simulink model "controller_8_9_2021_final"  (R2021a)
settings: Solver=ode23t  StartTime=0.0  StopTime=1.3  MaxStep=1  RelTol=1e-3  AbsTol=1e-3
model workspace (MAT data in the model file):
  T_ret = 0.5547
  T_standby = 0.2
values from neighbouring files (symbols this model uses):
  calculated_T_ramp = 0.012    [catapultScript_8_9_2021_final.m]
  calculated_T_ret = 0.07    [catapultScript_8_9_2021_final.m]
  calculated_W_cruise = 17.0    (= 17)    [catapultScript_8_9_2021_final.m]
  markerPosition = X_TARGET + L    [catapultScript_8_9_2021_final.m]
  speed_I = 1.2    [catapultScript_8_9_2021_final.m]
  speed_P = 2.6    [catapultScript_8_9_2021_final.m]
undefined symbols (not defined in the file or in its folder): ballNumber, torque, X, Y, Z
libraries: sm_lib x33, nesl_utility x11, ee_lib x6, fl_lib x5, pid_lib x2
(part 2 of 2)

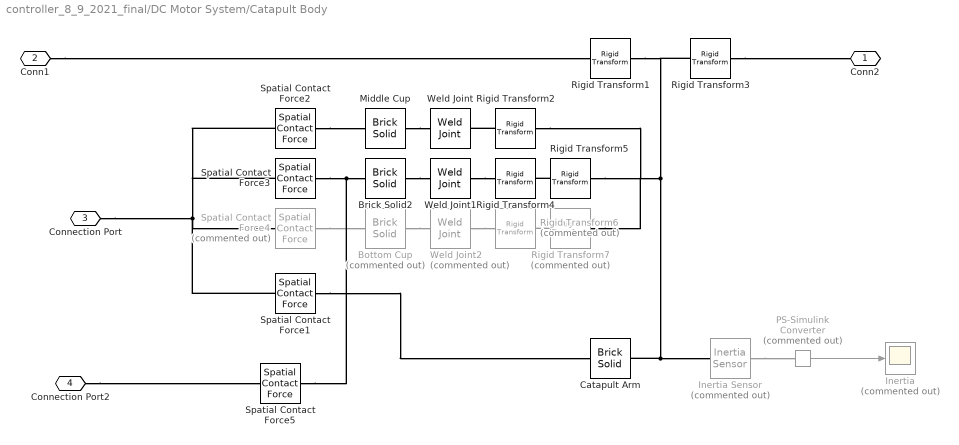
== system controller_8_9_2021_final/DC Motor System/Catapult Body ==
  Bottom Cup : sm_lib/Body Elements/Brick Solid  Commented=on  GraphicAmbientColor=[0.15 0.15 0.15 1.0]  BasedOnType=Density  BrickDimensions=[6 3 0.5]  BrickDimensionUnits=cm  CenterOfMass=[0 0 0]  CenterOfMassUnits=m  GraphicDiffuseColor=[0.0 0.8 0.6]  Density=1100  DensityUnits=kg/m^3  DoExposeReferenceFrame=on  GraphicEmissiveColor=[0.0 0.0 0.0 1.0]  ExportEntireGeometry=on  SerializedFrames=<Frames/>  MarkerShape=Sphere  MarkerSize=10  GraphicType=FromGeometry  InertiaType=CalculateFromGeometry  Mass=0  MassUnits=kg  MomentsOfInertia=[1 1 1]  MomentsOfInertiaUnits=kg*m^2  GraphicOpacity=1.0  ProductsOfInertia=[0 0 0]  ProductsOfInertiaUnits=kg*m^2  GraphicShininess=75  GraphicSpecularColor=[0.5 0.5 0.5 1.0]  GraphicVisPropType=SimpleVisualProperties
  Brick Solid2 : sm_lib/Body Elements/Brick Solid  GraphicAmbientColor=[0.15 0.15 0.15 1.0]  BasedOnType=Density  BrickDimensions=[6 3.5 0.5]  BrickDimensionUnits=cm  CenterOfMass=[0 0 0]  CenterOfMassUnits=m  GraphicDiffuseColor=[0.0 0.8 0.6]  Density=1100  DensityUnits=kg/m^3  DoExposeReferenceFrame=on  GraphicEmissiveColor=[0.0 0.0 0.0 1.0]  ExportEntireGeometry=on  SerializedFrames=<Frames/>  MarkerShape=Sphere  MarkerSize=10  GraphicType=FromGeometry  InertiaType=CalculateFromGeometry  Mass=1  MassUnits=kg  MomentsOfInertia=[1 1 1]  MomentsOfInertiaUnits=kg*m^2  GraphicOpacity=1.0  ProductsOfInertia=[0 0 0]  ProductsOfInertiaUnits=kg*m^2  GraphicShininess=75  GraphicSpecularColor=[0.5 0.5 0.5 1.0]  GraphicVisPropType=SimpleVisualProperties
  Catapult Arm : sm_lib/Body Elements/Brick Solid  GraphicAmbientColor=[0.15 0.15 0.15 1.0]  BasedOnType=Density  BrickDimensions=[27 2 2]  BrickDimensionUnits=cm  CenterOfMass=[0 0 0]  CenterOfMassUnits=m  GraphicDiffuseColor=[0.0 0.8 0.8]  Density=1100  DensityUnits=kg/m^3  DoExposeReferenceFrame=on  GraphicEmissiveColor=[0.0 0.0 0.0 1.0]  ExportEntireGeometry=on  SerializedFrames=<Frames/>  MarkerShape=Sphere  MarkerSize=10  GraphicType=FromGeometry  InertiaType=CalculateFromGeometry  Mass=1  MassUnits=kg  MomentsOfInertia=[2.291563*10^-3 0 0]  MomentsOfInertiaUnits=kg*m^2  GraphicOpacity=1.0  ProductsOfInertia=[0 0 0]  ProductsOfInertiaUnits=kg*m^2  GraphicShininess=75  GraphicSpecularColor=[0.5 0.5 0.5 1.0]  GraphicVisPropType=SimpleVisualProperties
  Inertia : Scope  Commented=on
  Inertia Sensor : sm_lib/Body Elements/Inertia Sensor  Commented=on  SensorExtent=BodyGroup  SpanWeldJoints=on  ExcludeGroundedBodies=off  MeasurementFrame=Attached  SenseMass=off  SenseCenterOfMass=off  SenseInertiaMatrix=off  SenseCenteredInertiaMatrix=off  SensePrincipalInertiaMatrix=on  SenseRotationMatrix=off  GraphicType=PrincipalInertiaFrame  PrincipalInertiaFrameSize=20  GraphicVisPropType=SimpleVisualProperties  GraphicDiffuseColor=[0.5 0.5 0.5]  GraphicSpecularColor=[0.5 0.5 0.5 1.0]  GraphicAmbientColor=[0.15 0.15 0.15 1.0]  GraphicEmissiveColor=[0.0 0.0 0.0 1.0]  GraphicShininess=75  GraphicOpacity=1.0
      settings: SourceProductBaseCode=MS
  Middle Cup : sm_lib/Body Elements/Brick Solid  GraphicAmbientColor=[0.15 0.15 0.15 1.0]  BasedOnType=Density  BrickDimensions=[6 6 1]  BrickDimensionUnits=cm  CenterOfMass=[0 0 0]  CenterOfMassUnits=m  GraphicDiffuseColor=[0.0 0.8 0.6]  Density=1100  DensityUnits=kg/m^3  DoExposeReferenceFrame=on  GraphicEmissiveColor=[0.0 0.0 0.0 1.0]  ExportEntireGeometry=on  SerializedFrames=<Frames/>  MarkerShape=Sphere  MarkerSize=10  GraphicType=FromGeometry  InertiaType=CalculateFromGeometry  Mass=1  MassUnits=kg  MomentsOfInertia=[1 1 1]  MomentsOfInertiaUnits=kg*m^2  GraphicOpacity=1.0  ProductsOfInertia=[0 0 0]  ProductsOfInertiaUnits=kg*m^2  GraphicShininess=75  GraphicSpecularColor=[0.5 0.5 0.5 1.0]  GraphicVisPropType=SimpleVisualProperties
  PS-Simulink Converter : nesl_utility/PS-Simulink Converter  Commented=on  PhysicalDomain=network_engine_domain  SubClassName=ps_output  LeftPortType=input  RightPortType=output  PseudoPeriodic=off  Frequencies=[]  Unit=inherit  AffineConversion=off
      settings: SourceProductBaseCode=PW,SS
  Rigid Transform1 : sm_lib/Frames and Transforms/Rigid Transform  TranslationMethod=StandardAxis  TranslationStandardOffset=-13.5  TranslationLengthUnit=cm  TranslationStandardAxis=+X  TranslationCartesianOffset=[0 0 0]  TranslationROffset=0  TranslationROffsetUnits=m  TranslationZOffset=0  TranslationZOffsetUnits=m  TranslationThetaOffset=0  TranslationThetaOffsetUnits=deg  RotationMethod=StandardAxis  RotationAngleUnits=deg  RotationStandardAxis=+Z  RotationAngle=forcedArmAngle  RotationArbitraryAxis=[0 0 1]  FollAlignAxisA=+X  BaseAlignAxisA=+Y  FollAlignAxisB=+Y  BaseAlignAxisB=+Z  RotationSequenceAxes=FollowerAxes  RotationSequence=XYX  RotationSequenceAngles=[0 0 0]  RotationSequenceAnglesUnits=deg  RotationMatrix=[1 0 0; 0 1 0; 0 0 1]
  Rigid Transform2 : sm_lib/Frames and Transforms/Rigid Transform  TranslationMethod=Cartesian  TranslationStandardOffset=7  TranslationLengthUnit=cm  TranslationStandardAxis=-X  TranslationCartesianOffset=[-11 0 -1]  TranslationROffset=0  TranslationROffsetUnits=m  TranslationZOffset=0  TranslationZOffsetUnits=m  TranslationThetaOffset=0  TranslationThetaOffsetUnits=deg  RotationMethod=StandardAxis  RotationAngleUnits=deg  RotationStandardAxis=+X  RotationAngle=90  RotationArbitraryAxis=[0 0 1]  FollAlignAxisA=+X  BaseAlignAxisA=+Y  FollAlignAxisB=+Y  BaseAlignAxisB=+Z  RotationSequenceAxes=FollowerAxes  RotationSequence=XYX  RotationSequenceAngles=[90 0 0]  RotationSequenceAnglesUnits=deg  RotationMatrix=[1 0 0; 0 1 0; 0 0 1]
  Rigid Transform3 : sm_lib/Frames and Transforms/Rigid Transform  TranslationMethod=StandardAxis  TranslationStandardOffset=7  TranslationLengthUnit=cm  TranslationStandardAxis=+X  TranslationCartesianOffset=[0 0 0]  TranslationROffset=0  TranslationROffsetUnits=m  TranslationZOffset=0  TranslationZOffsetUnits=m  TranslationThetaOffset=0  TranslationThetaOffsetUnits=deg  RotationMethod=None  RotationAngleUnits=deg  RotationStandardAxis=+Z  RotationAngle=30  RotationArbitraryAxis=[0 0 1]  FollAlignAxisA=+X  BaseAlignAxisA=+Y  FollAlignAxisB=+Y  BaseAlignAxisB=+Z  RotationSequenceAxes=FollowerAxes  RotationSequence=XYX  RotationSequenceAngles=[0 0 0]  RotationSequenceAnglesUnits=deg  RotationMatrix=[1 0 0; 0 1 0; 0 0 1]
  Rigid Transform4 : sm_lib/Frames and Transforms/Rigid Transform  TranslationMethod=Cartesian  TranslationStandardOffset=7  TranslationLengthUnit=cm  TranslationStandardAxis=-X  TranslationCartesianOffset=[-7 0 -1]  TranslationROffset=0  TranslationROffsetUnits=m  TranslationZOffset=0  TranslationZOffsetUnits=m  TranslationThetaOffset=0  TranslationThetaOffsetUnits=deg  RotationMethod=StandardAxis  RotationAngleUnits=deg  RotationStandardAxis=+X  RotationAngle=90  RotationArbitraryAxis=[0 0 1]  FollAlignAxisA=+X  BaseAlignAxisA=+Y  FollAlignAxisB=+Y  BaseAlignAxisB=+Z  RotationSequenceAxes=FollowerAxes  RotationSequence=XYX  RotationSequenceAngles=[90 0 0]  RotationSequenceAnglesUnits=deg  RotationMatrix=[1 0 0; 0 1 0; 0 0 1]
  Rigid Transform5 : sm_lib/Frames and Transforms/Rigid Transform  TranslationMethod=Cartesian  TranslationStandardOffset=7  TranslationLengthUnit=cm  TranslationStandardAxis=-X  TranslationCartesianOffset=[7 -13.2 -4]  TranslationROffset=0  TranslationROffsetUnits=m  TranslationZOffset=0  TranslationZOffsetUnits=m  TranslationThetaOffset=0  TranslationThetaOffsetUnits=deg  RotationMethod=RotationSequence  RotationAngleUnits=deg  RotationStandardAxis=+X  RotationAngle=90  RotationArbitraryAxis=[0 0 1]  FollAlignAxisA=+X  BaseAlignAxisA=+Y  FollAlignAxisB=+Y  BaseAlignAxisB=+Z  RotationSequenceAxes=FollowerAxes  RotationSequence=XYX  RotationSequenceAngles=[90 90 0]  RotationSequenceAnglesUnits=deg  RotationMatrix=[1 0 0; 0 1 0; 0 0 1]
  Rigid Transform6 : sm_lib/Frames and Transforms/Rigid Transform  Commented=on  TranslationMethod=Cartesian  TranslationStandardOffset=7  TranslationLengthUnit=cm  TranslationStandardAxis=-X  TranslationCartesianOffset=[-7 0 -1]  TranslationROffset=0  TranslationROffsetUnits=m  TranslationZOffset=0  TranslationZOffsetUnits=m  TranslationThetaOffset=0  TranslationThetaOffsetUnits=deg  RotationMethod=StandardAxis  RotationAngleUnits=deg  RotationStandardAxis=+X  RotationAngle=90  RotationArbitraryAxis=[0 0 1]  FollAlignAxisA=+X  BaseAlignAxisA=+Y  FollAlignAxisB=+Y  BaseAlignAxisB=+Z  RotationSequenceAxes=FollowerAxes  RotationSequence=XYX  RotationSequenceAngles=[90 0 0]  RotationSequenceAnglesUnits=deg  RotationMatrix=[1 0 0; 0 1 0; 0 0 1]
  Rigid Transform7 : sm_lib/Frames and Transforms/Rigid Transform  Commented=on  TranslationMethod=Cartesian  TranslationStandardOffset=7  TranslationLengthUnit=cm  TranslationStandardAxis=-X  TranslationCartesianOffset=[7 -2.4 -4]  TranslationROffset=0  TranslationROffsetUnits=m  TranslationZOffset=0  TranslationZOffsetUnits=m  TranslationThetaOffset=0  TranslationThetaOffsetUnits=deg  RotationMethod=RotationSequence  RotationAngleUnits=deg  RotationStandardAxis=+X  RotationAngle=90  RotationArbitraryAxis=[0 0 1]  FollAlignAxisA=+X  BaseAlignAxisA=+Y  FollAlignAxisB=+Y  BaseAlignAxisB=+Z  RotationSequenceAxes=FollowerAxes  RotationSequence=XYX  RotationSequenceAngles=[90 90 0]  RotationSequenceAnglesUnits=deg  RotationMatrix=[1 0 0; 0 1 0; 0 0 1]
  Spatial Contact Force1 : sm_lib/Forces and Torques/Spatial Contact Force  CoefficientOfDynamicFriction=0.3  CoefficientOfStaticFriction=0.5  SenseContactBaseRotation=off  SenseContactBaseTranslation=off  NormalDamping=1e3  NormalDampingUnits=N/(m/s)  SenseContactFollowerRotation=off  SenseContactFollowerTranslation=off  SenseContactSignal=off  NormalStiffness=1e6  NormalStiffnessUnits=N/m  FrictionalCriticalVelocity=1e-3  FrictionalCriticalVelocityUnits=m/s  ZeroCrossDetectContactStartAndEnd=off  FrictionType=SmoothStickSlip  SenseFrictionalForceMagnitude=off  SenseNormalForceMagnitude=off  NormalForceType=SmoothSpringDamper  SenseNormalVelocity=off  SenseSeparationDistance=off  SenseTangentialVelocity=off  SenseTangentialVelocityMagnitude=off  NormalTransitionRegionWidth=1e-4  NormalTransitionRegionWidthUnits=m
  Spatial Contact Force2 : sm_lib/Forces and Torques/Spatial Contact Force  CoefficientOfDynamicFriction=0.3  CoefficientOfStaticFriction=0.5  SenseContactBaseRotation=off  SenseContactBaseTranslation=off  NormalDamping=1e3  NormalDampingUnits=N/(m/s)  SenseContactFollowerRotation=off  SenseContactFollowerTranslation=off  SenseContactSignal=off  NormalStiffness=1e6  NormalStiffnessUnits=N/m  FrictionalCriticalVelocity=1e-3  FrictionalCriticalVelocityUnits=m/s  ZeroCrossDetectContactStartAndEnd=off  FrictionType=None  SenseFrictionalForceMagnitude=off  SenseNormalForceMagnitude=off  NormalForceType=SmoothSpringDamper  SenseNormalVelocity=off  SenseSeparationDistance=off  SenseTangentialVelocity=off  SenseTangentialVelocityMagnitude=off  NormalTransitionRegionWidth=1e-4  NormalTransitionRegionWidthUnits=m
  Spatial Contact Force3 : sm_lib/Forces and Torques/Spatial Contact Force  CoefficientOfDynamicFriction=0.3  CoefficientOfStaticFriction=0.5  SenseContactBaseRotation=off  SenseContactBaseTranslation=off  NormalDamping=1e3  NormalDampingUnits=N/(m/s)  SenseContactFollowerRotation=off  SenseContactFollowerTranslation=off  SenseContactSignal=off  NormalStiffness=1e6  NormalStiffnessUnits=N/m  FrictionalCriticalVelocity=1e-3  FrictionalCriticalVelocityUnits=m/s  ZeroCrossDetectContactStartAndEnd=off  FrictionType=None  SenseFrictionalForceMagnitude=off  SenseNormalForceMagnitude=off  NormalForceType=SmoothSpringDamper  SenseNormalVelocity=off  SenseSeparationDistance=off  SenseTangentialVelocity=off  SenseTangentialVelocityMagnitude=off  NormalTransitionRegionWidth=1e-4  NormalTransitionRegionWidthUnits=m
  Spatial Contact Force4 : sm_lib/Forces and Torques/Spatial Contact Force  Commented=on  CoefficientOfDynamicFriction=0.3  CoefficientOfStaticFriction=0.5  SenseContactBaseRotation=off  SenseContactBaseTranslation=off  NormalDamping=1e3  NormalDampingUnits=N/(m/s)  SenseContactFollowerRotation=off  SenseContactFollowerTranslation=off  SenseContactSignal=off  NormalStiffness=1e6  NormalStiffnessUnits=N/m  FrictionalCriticalVelocity=1e-3  FrictionalCriticalVelocityUnits=m/s  ZeroCrossDetectContactStartAndEnd=off  FrictionType=SmoothStickSlip  SenseFrictionalForceMagnitude=off  SenseNormalForceMagnitude=off  NormalForceType=SmoothSpringDamper  SenseNormalVelocity=off  SenseSeparationDistance=off  SenseTangentialVelocity=off  SenseTangentialVelocityMagnitude=off  NormalTransitionRegionWidth=1e-4  NormalTransitionRegionWidthUnits=m
  Spatial Contact Force5 : sm_lib/Forces and Torques/Spatial Contact Force  CoefficientOfDynamicFriction=0.3  CoefficientOfStaticFriction=0.5  SenseContactBaseRotation=off  SenseContactBaseTranslation=off  NormalDamping=1e3  NormalDampingUnits=N/(m/s)  SenseContactFollowerRotation=off  SenseContactFollowerTranslation=off  SenseContactSignal=off  NormalStiffness=1e6  NormalStiffnessUnits=N/m  FrictionalCriticalVelocity=1e-3  FrictionalCriticalVelocityUnits=m/s  ZeroCrossDetectContactStartAndEnd=off  FrictionType=SmoothStickSlip  SenseFrictionalForceMagnitude=off  SenseNormalForceMagnitude=off  NormalForceType=SmoothSpringDamper  SenseNormalVelocity=off  SenseSeparationDistance=off  SenseTangentialVelocity=off  SenseTangentialVelocityMagnitude=off  NormalTransitionRegionWidth=1e-4  NormalTransitionRegionWidthUnits=m
  Weld Joint : sm_lib/Joints/Weld Joint  JointMode=Normal  SenseConstraintForce=off  SenseConstraintForceX=off  SenseConstraintForceY=off  SenseConstraintForceZ=off  SenseConstraintTorque=off  SenseConstraintTorqueX=off  SenseConstraintTorqueY=off  SenseConstraintTorqueZ=off  SenseTotalForce=off  SenseTotalForceX=off  SenseTotalForceY=off  SenseTotalForceZ=off  SenseTotalTorque=off  SenseTotalTorqueX=off  SenseTotalTorqueY=off  SenseTotalTorqueZ=off  CompositeWrenchDir=FollowerOnBase  CompositeWrenchFrame=BaseFrame
  Weld Joint1 : sm_lib/Joints/Weld Joint  JointMode=Normal  SenseConstraintForce=off  SenseConstraintForceX=off  SenseConstraintForceY=off  SenseConstraintForceZ=off  SenseConstraintTorque=off  SenseConstraintTorqueX=off  SenseConstraintTorqueY=off  SenseConstraintTorqueZ=off  SenseTotalForce=off  SenseTotalForceX=off  SenseTotalForceY=off  SenseTotalForceZ=off  SenseTotalTorque=off  SenseTotalTorqueX=off  SenseTotalTorqueY=off  SenseTotalTorqueZ=off  CompositeWrenchDir=FollowerOnBase  CompositeWrenchFrame=BaseFrame
  Weld Joint2 : sm_lib/Joints/Weld Joint  Commented=on  JointMode=Normal  SenseConstraintForce=off  SenseConstraintForceX=off  SenseConstraintForceY=off  SenseConstraintForceZ=off  SenseConstraintTorque=off  SenseConstraintTorqueX=off  SenseConstraintTorqueY=off  SenseConstraintTorqueZ=off  SenseTotalForce=off  SenseTotalForceX=off  SenseTotalForceY=off  SenseTotalForceZ=off  SenseTotalTorque=off  SenseTotalTorqueX=off  SenseTotalTorqueY=off  SenseTotalTorqueZ=off  CompositeWrenchDir=FollowerOnBase  CompositeWrenchFrame=BaseFrame
  Conn2 : PMIOPort  Side=Right
  Conn1 : PMIOPort  Port=2  Side=Left
  Connection Port : PMIOPort  Port=3  Side=Left
  Connection Port2 : PMIOPort  Port=4  Side=Left
  wires:
  PS-Simulink Converter/1 -> Inertia/1
  connections:
  Rigid Transform7/LConn1 -- Rigid Transform6/RConn1
  Weld Joint2/RConn1 -- Rigid Transform6/LConn1
  Bottom Cup/RConn1 -- Weld Joint2/LConn1
  Rigid Transform5/LConn1 -- Rigid Transform4/RConn1
  Weld Joint1/RConn1 -- Rigid Transform4/LConn1
  Brick Solid2/RConn1 -- Weld Joint1/LConn1
  Middle Cup/RConn1 -- Weld Joint/LConn1
  Spatial Contact Force1/RConn1 -- Catapult Arm/LConn1
  Rigid Transform3/LConn1 -- Conn2/RConn1
  Conn1/RConn1 -- Rigid Transform1/RConn1
  Rigid Transform7/RConn1 -- Rigid Transform5/RConn1 -- Rigid Transform2/RConn1 -- Rigid Transform1/LConn1 -- Rigid Transform3/RConn1 -- Catapult Arm/RConn1 -- Inertia Sensor/LConn1
  Rigid Transform2/LConn1 -- Weld Joint/RConn1
  Inertia Sensor/RConn1 -- PS-Simulink Converter/LConn1
  Connection Port/RConn1 -- Spatial Contact Force3/LConn1 -- Spatial Contact Force2/LConn1 -- Spatial Contact Force1/LConn1 -- Spatial Contact Force4/LConn1
  Spatial Contact Force4/RConn1 -- Bottom Cup/LConn1
  Spatial Contact Force3/RConn1 -- Spatial Contact Force5/RConn1 -- Brick Solid2/LConn1
  Spatial Contact Force2/RConn1 -- Middle Cup/LConn1
  Connection Port2/RConn1 -- Spatial Contact Force5/LConn1

== matlab function controller_8_9_2021_final/MATLAB Function ==
  data: t input; ballNumber input; T_standby input; controlSwitch output; stage0Done input; T_ramp input; T_ret input; T_fin input; W_cruise input; Q_ret input; S3_ACCEL input; q_d output; dq_d output; d2q_d output
%References
% https://www.mathworks.com/help/matlab/ref/function.html
% Dr. Moallem's code - checked inputs & outputs initially,used inverse method for the quintic controller, and compared
% sections of my written code with his



%do we want to use T_ret or Theta_ret to switch stage?

function [controlSwitch, q_d, dq_d, d2q_d] = catapult_control( t,ballNumber,T_standby,stage0Done,T_ramp, T_ret, T_fin, W_cruise, Q_ret,S3_ACCEL) 
%function [controlSwitch, e_sc, e_pc, q_d, dq_d, d2q_d] = catapult_control( t,stage0Done,T_ramp, T_ret, T_fin, W_cruise, Q_ret, tau_scommand, tau_pcommand, theta, w, S3_ACCEL) 
%^ old header using tau,tau_scommand, tau_pcommand


controlSwitch = 0; %0 -> speed controller, 1 -> position controller

if stage0Done == 1
    t = t - T_standby;
end

%Stage 0 (Move to Starting Position: Q_ret)
% if stage0Done ~= 1 && t < T_standby && t < 0.8 && ballNumber == 1
%     %tau = tau_scommand; %based on speed control output
%     d2q_d = 2/0.8; %0.8s rise tarm hardcoded
%     dq_d = 2*t/0.8;
%      q_d = 0.5*d2q_d*(t^2);
%     %e_sc = dq_d - w;
%     %e_pc = 0; %since we don't need to change the system based on it
if stage0Done ~= 1 && t < T_standby
    controlSwitch = 1;
    q_d = Q_ret;
    dq_d = 0;
    d2q_d = 0;
    %e_sc = dq_d - w;
    %e_pc = q_d - theta;
    %tau = tau_pcommand;


%Stage 1 (Ramp up phase)
elseif t > 0 && t < T_ramp %Stage 1
controlSwitch = 0;    
    %tau = tau_scommand; %based on speed control output
    d2q_d = W_cruise/T_ramp;
    dq_d = W_cruise*t/T_ramp;
     q_d = 0.5*d2q_d*(t^2)+Q_ret;
    %e_sc = dq_d - w;
    %e_pc = 0; %since we don't need to change the system based on it

%Stage 2 (Constant Speed phase)
elseif t >= T_ramp && t < T_ret %Stage 2
    controlSwitch = 0;      
    %tau = tau_scommand; %based on speed control output
    q_d = 0.5*(W_cruise/T_ramp)*(T_ramp^2) + W_cruise*(t-T_ramp)+Q_ret; 
    dq_d = W_cruise;
    d2q_d = 0;
    %e_sc = W_cruise - w;
    %e_pc = 0; %since don't need to change the system based on it

 

%Stage 3 (Return Phase)
elseif t >= T_ret && t < T_fin %Stage 3
    controlSwitch = 1;   
    AT = T_fin - T_ret;
    %calculating qs
    q0 = 0.5*(W_cruise/T_ramp)*(T_ramp^2) + W_cruise*(T_ret - T_ramp)+Q_ret; %0.5*W_cruise*(T_ramp); %%It seems he already had the angle at this point known and hardcoded 

    q1 = W_cruise;
    q2 = 0.5*S3_ACCEL;
    
    ii= inv([AT^3 AT^4 AT^5; 3*AT^2 4*AT^3 5*AT^4; 6*AT 12*AT^2 20*AT^3])*[-(q0-Q_ret)-q1*AT-q2*AT^2; -q1-2*q2*AT; -2*q2];
    q3 = ii(1);
    q4 = ii(2);
    q5 = ii(3);
    %q5 = -(q0 + q1 - 0.3*q1*(T_fin - T_ret) - 0.6*q2*(T_fin - T_ret) + 1.033*q2*((T_fin - T_ret)^2))/(6.5*((T_fin - T_ret)^5));
    %q4 = -(q1 + 2*q2 + q2*((T_fin - T_ret) + 15*q5*((T_fin - T_ret)^4)))/(10*((T_fin - T_ret)^3));
    %q3 = (2*q2 + 12*q4*((T_fin - T_ret)^2) + 20*q5*((T_fin - T_ret)^3))/(6*(T_fin - T_ret));
    
    %main calculations
    AT = t - T_ret;
        
    q_d = q0 + q1*AT + q2*(AT^2) + q3*(AT^3) + q4*(AT^4) + q5*(AT^5);
    dq_d = q1 + 2*q2*AT + 3*q3*(AT^2) + 4*q4*(AT^3) + 5*q5*(AT^4);
    d2q_d = 2*q2 + 6*q3*AT + 12*q4*(AT^2) + 20*q5*(AT^3);
    %e_sc = dq_d - w;
    %e_pc = q_d - theta;
    %tau = tau_pcommand;  

else
    controlSwitch = 1;   
    %throw over, arm should be stationary
    q_d = Q_ret;
    dq_d = 0;
    d2q_d = 0;
    %e_sc = dq_d - w;
    %e_pc = q_d - theta;
    %tau = tau_pcommand;
    
end


end
